simulink model "power_windgen"  (Simulink 6.0)
settings: Solver=ode23tb  StartTime=0.0  StopTime=5  RelTol=1e-4
InitFcn:
  | load power_windgen_init
undefined symbols (not defined in the file or in its folder): DiscIntNeverNeededParam, psbwindgen_char
libraries: powerlib x43, powerlib_extras x6
Description:
  | The Model initialization function Callback automatically
  | 
  | loads the initial states vector xInitial and the wind turbine
  | 
  | characteristics. The initial conditions are stored in the
  | 
  | power_windgen_init.mat file.
settings Model: Creator=Richard Gagnon, IREQ  LastModifiedBy=batserve  ExtModeAutoUpdateStatusClock=off  ProdHWDeviceType=Specified
settings DataIOCC: LimitDataPoints=off  LoadInitialState=on  SaveOutput=off  SignalLoggingName=sigsOut
settings OptimizationCC: BlockReduction=off  BooleanDataType=off
settings DebuggingCC: CheckExecutionContextPreStartOutputMsg=on  CheckExecutionContextRuntimeOutputMsg=on  SolverPrmCheckMsg=none
settings HardwareCC: ProdBitPerShort=32  ProdBitPerInt=16  ProdHWDeviceType=Specified  TargetUnknown=on

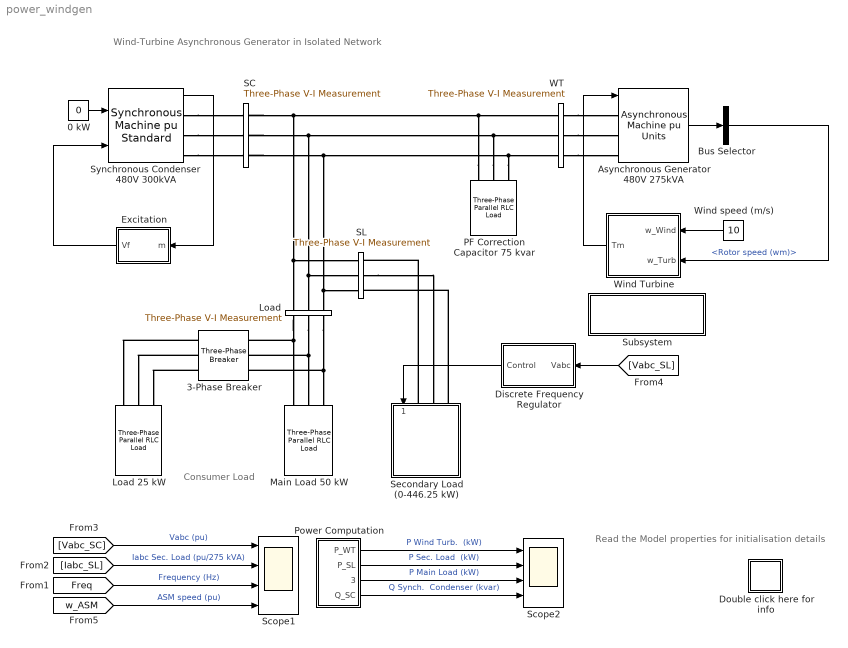
== system power_windgen ==
  note: Wind-Turbine Asynchronous Generator in Isolated Network
  note: Consumer Load
  note: Read the Model properties
      | for initialisation details
  0 kW : Constant  Value=0
  3-Phase Breaker : powerlib/Elements/Three-Phase Breaker  Orientation=left  InitialState=open  SwitchA=on  SwitchB=on  SwitchC=on  SwitchTimes=[0.2]  External=off  BreakerResistance=0.001  SnubberResistance=1e6  SnubberCapacitance=inf  Measurements=None
      settings: AttributesFormatString=\n
  Asynchronous Generator 480V 275kVA : powerlib/Machines/Asynchronous Machine pu Units  PresetModel=No  ShowDetailedParameters=on  RotorType=Squirrel-cage  ReferenceFrame=Rotor  NominalParameters=[ 275e3, 480, 60 ]  Stator=[ 0.016,0.06]  Rotor=[ 0.015,0.06]  Lm=3.5  Mechanical=[ 2,0,2 ]  InitialConditions=[-8.89496e-048 0 0.280896 0.280896 0.280896 -89.7425 150.258 30.2575]  Units=0  LoadFlowParameters=0
      settings: AttributesFormatString=\n
  Bus Selector : BusSelector  DialogController=Simulink.DDGSource_Bus  OutputSignals=Mechanical.Rotor speed (wm)
  Discrete Frequency Regulator : Subsystem  Orientation=left  mask(Discrete Frequency Regulator){Freq_ref=60, gains_regulator=[255 30], Vpp_nom=480, Ts=200e-6}
      mask prompts: Freq_ref "Reference frequency (Hz):"; gains_regulator "Regulator gains  [Kp Kd]:"; Vpp_nom "Phase to phase voltage (Vrms):"; Ts "Sample time (s):"
      mask help:
      | Input : phase to ground voltages
      |
      | Output : 24 logical signals for the control of the dump load
      mask init:
      | Vbase=Vpp_nom/sqrt(3);
      | Kp=gains_regulator(1);
      | Kd=gains_regulator(2);
  Double click here for info : Subsystem
      mask Display: disp('?')
  Excitation : Subsystem  Orientation=left
  Load : powerlib/Measurements/Three-Phase V-I Measurement  Orientation=down  VoltageMeasurement=phase-to-ground  SetLabelV=on  LabelV=Vabc_Load  Vpu=on  Vbase=480  CurrentMeasurement=yes  SetLabelI=on  LabelI=Iabc_Load  Ipu=on  Pbase=275e3  OutputType=Magnitude  PhasorSimulation=off  PSBequivalent=0
  Load 25 kW : powerlib/Elements/Three-Phase Parallel RLC Load  Orientation=down  PhysicalDomain=powersysdomain  SubClassName=unknown  LeftPortType=p1  RightPortType=p1  LConnTagsString=A|B|C  Configuration=Y (grounded)  NominalVoltage=480  NominalFrequency=60  ActivePower=25e3  InductivePower=0  CapacitivePower=0  Measurements=None
  Main Load 50 kW : powerlib/Elements/Three-Phase Parallel RLC Load  Orientation=down  PhysicalDomain=powersysdomain  SubClassName=unknown  LeftPortType=p1  RightPortType=p1  LConnTagsString=A|B|C  Configuration=Y (grounded)  NominalVoltage=480  NominalFrequency=60  ActivePower=50e3  InductivePower=0  CapacitivePower=0  Measurements=None
  PF Correction Capacitor 75 kvar : powerlib/Elements/Three-Phase Parallel RLC Load  Orientation=down  PhysicalDomain=powersysdomain  SubClassName=unknown  LeftPortType=p1  RightPortType=p1  LConnTagsString=A|B|C  Configuration=Delta  NominalVoltage=480  NominalFrequency=60  ActivePower=0  InductivePower=0  CapacitivePower=75e3  Measurements=None
  Power Computation : Subsystem
  SC : powerlib/Measurements/Three-Phase V-I Measurement  VoltageMeasurement=phase-to-ground  SetLabelV=on  LabelV=Vabc_SC  Vpu=on  Vbase=480  CurrentMeasurement=yes  SetLabelI=on  LabelI=Iabc_SC  Ipu=on  Pbase=300e3  OutputType=Magnitude  PhasorSimulation=off  PSBequivalent=0
  SL : powerlib/Measurements/Three-Phase V-I Measurement  VoltageMeasurement=phase-to-ground  SetLabelV=on  LabelV=Vabc_SL  Vpu=on  Vbase=480  CurrentMeasurement=yes  SetLabelI=on  LabelI=Iabc_SL  Ipu=on  Pbase=275e3  OutputType=Magnitude  PhasorSimulation=off  PSBequivalent=0
  Scope1 : Scope  NumInputPorts=4
      settings: TimeRange=5  YMin=-1.25~-0.75~59.8~1.008  YMax=1.25~0.75~60.1~1.013  SaveName=Vabc
  Scope2 : Scope  NumInputPorts=4
      settings: TimeRange=5  YMin=180~100~50~18  YMax=240~160~80~30  SaveName=Power  DataFormat=Array
  Secondary Load (0-446.25 kW) : Subsystem  Orientation=down  mask(8-step Variable Load){Vphase_phase_lissage=480, Freq=60, P_lissage_min=1.75e3, Pin_3phase=50e3}
      mask prompts: Vphase_phase_lissage "Nominal L-L voltage (Vrms):"; Freq "Nominal frequency (Hz):"; P_lissage_min "Power per step Pstep (W):"; Pin_3phase "Initial power  (W) :"
      mask help:
      | This block implements a variable, three-phase resistive load. The load variation uses an eight-bit binary progression so that the load power can be varied by steps from 0 to 255*Pstep.
      |
      | The eight three-phase resistors are connected in series with ideal switches simulating forced-commutated power electronic switches.
      |
      | The Pulses input is a vector containing the eight bits (0/1) controlling the eight three-phase switches. First value is the less significant bit.
      mask init:
      | Ron_switch=1e-6;
      | Rs_snubber=inf;
      | Cs_snubber=0;
      | n_niveaux=8;
      | Pmax=((2^n_niveaux)-1)*P_lissage_min;
      | Pin_normalise=min([(Pin_3phase/Pmax)*((2^n_niveaux)-1) ((2^n_niveaux)-1)]);
      | discret1=pow2(0:-1:-(n_niveaux-1))*Pin_normalise;
      | discret2=floor(discret1);
      | Status=rem(discret2,2);
  Subsystem : Subsystem
      settings: OpenFcn=open('psbwindgen_turb.fig')
      mask Display: disp('Double click to display\nTurbine characteristics')
  Synchronous Condenser  480V 300kVA : powerlib/Machines/Synchronous Machine pu Standard  PresetModel=No  ShowDetailedParameters=on  RotorType=Salient-pole  NominalParameters=[ 300e3 480 60 ]  Reactances1=[ 3.23, 0.21, 0.15, 2.79, 1.03, 0.37, 0.09 ]  Reactances2=[ 3.23, 0.21, 0.15, 2.79, 0.37, 0.09]  dAxisTimeConstants=Open-circuit  qAxisTimeConstants=Open-circuit  TimeConstants1="[ 1.7  0.008  0.004]"  TimeConstants2=[ 1.7, 0.008, 0.213, 0.004 ]  TimeConstants3="[  1.7 0.008 0.051266  ]"  TimeConstants4=[ 8.0, 0.03, 0.3371, 0.0295 ]  TimeConstants5="[ 0.08  0.019  0.004 ]"  TimeConstants6=[ 1.3201, 0.023, 1.0, 0.07 ]  TimeConstants7="[  0.08  0.019 0.051266  ]"  TimeConstants8=[ 1.3201, 0.0231, 0.3371, 0.0295 ]  StatorResistance=0.017  Mechanical=[ 1, 0, 2 ]  InitialConditions=[0 -89.2146 0.827 0.827 0.827 -86.4 153.6 33.6 2.71455]  SetSaturation=off  Saturation=[0.6404,0.7127,0.8441,0.9214,0.9956,1.082,1.19,1.316,1.457;0.7,0.7698,0.8872,0.9466,0.9969,1.046,1.1,1.151,1.201]  Units=0.5  LoadFlowParameters=[2 0 0 0 0]
      settings: AttributesFormatString=\n\n
  WT : powerlib/Measurements/Three-Phase V-I Measurement  VoltageMeasurement=phase-to-ground  SetLabelV=on  LabelV=Vabc_WT  Vpu=on  Vbase=480  CurrentMeasurement=yes  SetLabelI=on  LabelI=Iabc_WT  Ipu=on  Pbase=275e3  OutputType=Magnitude  PhasorSimulation=off  PSBequivalent=0
  Wind Turbine : Subsystem  Orientation=left
  Wind speed (m/s) : Constant  Orientation=left  Value=10
  wires:
  [Freq] -> Scope1/3  "Frequency (Hz)"
  [Vabc_SC] -> Scope1/1  "Vabc (pu)"
  [Iabc_SL] -> Scope1/2  "Iabc Sec. Load (pu/275 kVA)"
  Wind speed (m/s)/1 -> Wind Turbine/1(w_Wind)
  [Vabc_SL] -> Discrete Frequency Regulator/1(Vabc)
  Power Computation/1(P_WT) -> Scope2/1  "P Wind Turb.  (kW)"
  Power Computation/2(P_SL) -> Scope2/2  "P Sec. Load  (kW)"
  Power Computation/3(P_Load) -> Scope2/3  "P Main Load (kW)"
  Power Computation/4(Q_SC) -> Scope2/4  "Q Synch.  Condenser (kvar)"
  Discrete Frequency Regulator/1(Control) -> Secondary Load (0-446.25 kW)/1(Control)
  [w_ASM] -> Scope1/4  "ASM speed (pu)"
  0 kW/1 -> Synchronous Condenser  480V 300kVA/1
  Synchronous Condenser  480V 300kVA/1 -> Excitation/1(m)
  Excitation/1(Vf) -> Synchronous Condenser  480V 300kVA/2
  Asynchronous Generator 480V 275kVA/1 -> Bus Selector/1
  Wind Turbine/1(Tm) -> Asynchronous Generator 480V 275kVA/1
  Bus Selector/1 -> Wind Turbine/2(w_Turb)  "<Rotor speed (wm)>"
  connections:
  Load/RConn3 -- Main Load 50 kW/LConn3 -- 3-Phase Breaker/LConn3
  Load/RConn1 -- Main Load 50 kW/LConn1 -- 3-Phase Breaker/LConn1
  Load/RConn2 -- Main Load 50 kW/LConn2 -- 3-Phase Breaker/LConn2
  WT/RConn1 -- Asynchronous Generator 480V 275kVA/LConn1
  WT/RConn2 -- Asynchronous Generator 480V 275kVA/LConn2
  WT/RConn3 -- Asynchronous Generator 480V 275kVA/LConn3
  Synchronous Condenser  480V 300kVA/RConn1 -- SC/LConn1
  Synchronous Condenser  480V 300kVA/RConn2 -- SC/LConn2
  Synchronous Condenser  480V 300kVA/RConn3 -- SC/LConn3
  PF Correction Capacitor 75 kvar/LConn1 -- SC/RConn1 -- SL/LConn1 -- Load/LConn1 -- WT/LConn1
  PF Correction Capacitor 75 kvar/LConn2 -- SC/RConn2 -- SL/LConn2 -- Load/LConn2 -- WT/LConn2
  PF Correction Capacitor 75 kvar/LConn3 -- SC/RConn3 -- SL/LConn3 -- Load/LConn3 -- WT/LConn3
  3-Phase Breaker/RConn1 -- Load 25 kW/LConn1
  3-Phase Breaker/RConn2 -- Load 25 kW/LConn2
  3-Phase Breaker/RConn3 -- Load 25 kW/LConn3
  Secondary Load (0-446.25 kW)/LConn1 -- SL/RConn1
  SL/RConn2 -- Secondary Load (0-446.25 kW)/LConn2
  Secondary Load (0-446.25 kW)/LConn3 -- SL/RConn3

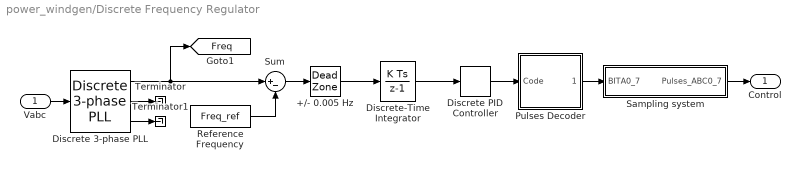
== system power_windgen/Discrete Frequency Regulator ==
  Vabc : Inport  Port=1  LatchInput=off
  +/- 0.005 Hz : DeadZone  LowerValue=-0.005  UpperValue=0.005  SaturateOnIntegerOverflow=on
  Discrete 3-phase PLL : powerlib_extras/Discrete  Control Blocks/Discrete 3-phase PLL  Fmin=45  Par_Init=[0 Freq_ref]  ParK=[60 1400]  Ts=Ts
  Discrete PID Controller : powerlib_extras/Discrete  Control Blocks/Discrete PID Controller  Kp=Kp  Ki=0  Kd=Kd  TcD=0.5e-3  Par_Limits=[255 0]  Init=0  Ts=Ts
  Discrete-Time Integrator : DiscreteIntegrator  SampleTime=Ts  LimitOutput=on  UpperSaturationLimit=1  LowerSaturationLimit=0  ICPrevOutput=DiscIntNeverNeededParam  ICPrevScaledInput=DiscIntNeverNeededParam
  Pulses Decoder : Subsystem  mask(Pulses Decoder){n=8}
      mask prompts: n "Number of bits to decode:"
      mask help:
      | Decode the scalar input 'Code' into a vector output 'Pulses' based on  the specified number of bits to decode.
      | (Element 1 of vector output = least significant bit)
  Reference Frequency : Constant  Value=Freq_ref
  Sampling system : Subsystem
  Sum : Sum  Inputs=|+-  SaturateOnIntegerOverflow=on  InputSameDT=on
  Terminator : Terminator
  Terminator1 : Terminator
  Control : Outport
  tag scope: Freq=global
  wires:
  Vabc/1 -> Discrete 3-phase PLL/1
  Discrete 3-phase PLL/3 -> Terminator1/1
  Discrete 3-phase PLL/2 -> Terminator/1
  Sampling system/1(Pulses_ABC0_7) -> Control/1
  Discrete-Time Integrator/1 -> Discrete PID Controller/1
  Reference Frequency/1 -> Sum/2
  Discrete PID Controller/1 -> Pulses Decoder/1(Code)
  Sum/1 -> +/- 0.005 Hz/1
  Pulses Decoder/1(Pulses) -> Sampling system/1(BITA0_7)
  +/- 0.005 Hz/1 -> Discrete-Time Integrator/1
  Discrete 3-phase PLL/1 -> Sum/1, [Freq]

== system power_windgen/Double click here for info ==
  note: [1] R. Gagnon, B. Saulnier, G. Sybille, P. Giroux; "Modeling of a Generic High-Penetration No-Storage Wind-Diesel System Using Matlab/Power System Blockset"
      | 2002 Global Windpower Conference, April 2002, Paris, France
      | [2] B. Saulnier, A.O. Barry, B. Dube, R. Reid; "Design and Development of a Regulation and Control System for the High-Penetration No-Storage Wind/Diesel
      | Scheme" European Community Wind Energy Conference 88, 6-10 june 1988, Herning, Denmark
      | [3] L. Mott (NPS), B. Saulnier (IREQ) " Commercial Wind-Diesel Project, St. Paul Island, Alaska" 14th Prime Power Diesel Inter-Utility Conference,
      | May 28-June 2, Winnipeg, Manitoba, Canada
  note: References
  note: For the demo, the wind speed (10m/s) is such that the wind turbine produces enough power to supply the load. The diesel-generator (not simulated) is stopped
      | and the synchronous machine operates as a synchronous condenser with its mechanical power input (Pm) set at zero.
      | The demo illustrates the dynamic performance of the frequency regulation system when an additional 25 kW customer load is switched on.
      |
      | Start simulation and observe voltages, currents, powers, asynchronous machine speed and system frequency on the two scopes.
      | Initial conditions (xInitial vector) have been automatically loaded in your workspace so that simulation starts in steady state.
      |
      | As the asynchronous machine operates in generator mode, its speed is slightly above the synchronous speed (1.011 pu).
      | According to turbine characteristics, for a 10m/s wind speed, the turbine output power is 0.75 pu (206 kW). Because of the asynchronous machine losses,
      | the wind turbine produces 200 kW. As the main load is 50 kW, the secondary load absorbs 150 kW to maintain a constant 60 Hz frequency.
      | At t=0.2 s, the additional load of 25 kW is switched on. The frequency  momentarily drops to 59.85 Hz and the frequency regulator reacts to reduce the power
      | absorbed by the secondary load in order to bring the frequency back to 60 Hz. Voltage stays at 1 pu and no flicker is observed.
  note: R. Reid, B. Saulnier, R. Gagnon; Hydro-Quebec (IREQ)
  note: A generic model of the High-Penetration, No Storage, Wind-Diesel (HPNSWD) system is presented in this demo [1].
      | This technology was developed by Hydro-Quebec to reduce the cost of supplying electricity in remote northern communities[2].
      | The optimal wind penetration (installed wind capacity/peak electrical demand) for this system depends on the site delivery cost of fuel
      | and available wind resource. The first commercial application of HPNSWD technology was commissioned in 1999 by Northern Power Systems (Vermont,USA)
      | on St. Paul Island, Alaska [3]. The HPNSWD system presented in this demo uses a 480 V, 300 kVA synchronous machine, a wind turbine driving
      | a 480 V, 275 kVA induction generator, a 50 kW customer load and a variable secondary load (0 to 446.25 kW).
      |
      | At low wind speeds both the induction generator and the diesel-driven synchronous generator are required to feed the load.
      | When the wind power exceeds the load demand, it is possible to shut down the diesel-generator. In this all-wind mode, the synchronous machine
      | is used as a synchronous condenser and its excitation system controls the grid voltage at its nominal value.
      | A secondary load bank is used to regulate the system frequency by absorbing the wind power exceeding consumer demand.
      |
      | The Wind Turbine block uses a 2-D Lookup Table to compute the turbine torque output (Tm) as a function of wind speed (w_Wind) and turbine speed (w_Turb).
      | When you opened this demo, the Pm(w_Wind, w_Turb) characteristics was automatically loaded in your workspace (psbwindgen_char array).
      | To display the turbine characteristics, double click on the block located below the Wind Turbine block.
      |
      | The Secondary Load block consists of eight sets of three-phase resistors connected in series with GTO thyristor switches.
      | The nominal power of each set follows a binary progression so that the load can be varied from 0 to 446.25 kW by steps of 1.75kW.
      | GTOs are simulated by ideal switches.
      |
      | The frequency is controlled by the Discrete Frequency Regulator block. This controller uses a standard three-phase Phase Locked Loop (PLL) system to
      | measure the system frequency. The measured frequency is compared to the reference frequency (60 Hz) to obtain the frequency error.
      | This error is integrated to obtain the phase error. The phase error is then used  by a Proportional-Differential (PD) controller to produce an output signal
      | representing the required secondary load power. This signal is converted to an 8-bit digital signal controlling switching of the eight three-phase secondary loads.
      | In order to minimize voltage disturbances, switching is performed at zero crossing of voltage.
  note: Wind-Turbine Asynchronous Generator in Isolated Network
  note: Circuit Description
  note: Demonstration

== system power_windgen/Excitation ==
  m : Inport  Orientation=left  Port=1  LatchInput=off
  Bus Selector1 : BusSelector  Orientation=left  DialogController=Simulink.DDGSource_Bus  OutputSignals="dq0 components.Stator voltage  vd (pu),dq0 components.Stator voltage  vq (pu)"
  Constant3 : Constant  Orientation=left
  Excitation System : powerlib/Machines/Excitation System  Orientation=left  tr=20e-3  reg=[ 300, 0.001 ]  exc=[ 1, 0 ]  tgr=[ 0, 0 ]  damp=[ 0.001, 0.1 ]  sat=[ 0, 0 ]  lim=[ -11.5, 11.5, 0 ]  v0=[1,2.71455]
  Ground : Ground  Orientation=left
  Vf : Outport  Orientation=left
  wires:
  Constant3/1 -> Excitation System/1
  Ground/1 -> Excitation System/4
  m/1 -> Bus Selector1/1
  Excitation System/1 -> Vf/1
  Bus Selector1/1 -> Excitation System/2  "<Stator voltage  vd (pu)>"
  Bus Selector1/2 -> Excitation System/3  "<Stator voltage  vq (pu)>"

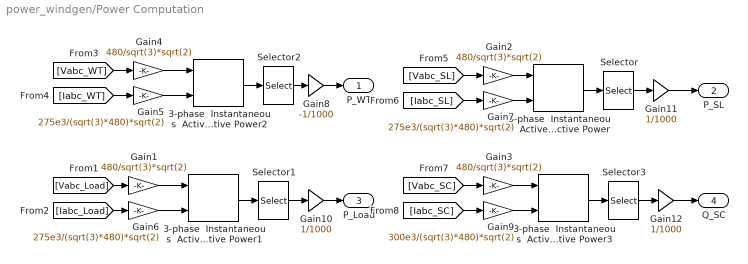
== system power_windgen/Power Computation ==
  3-phase  Instantaneous  Active & Reactive Power{,1..3} (4 alike) : powerlib_extras/Measurements/3-phase  Instantaneous  Active & Reactive Power
  Gain{1..4} (4 alike) : Gain  Gain=480/sqrt(3)*sqrt(2)  SaturateOnIntegerOverflow=on
  Gain10 : Gain  Gain=1/1000  SaturateOnIntegerOverflow=on
  Gain11 : Gain  Gain=1/1000  SaturateOnIntegerOverflow=on
  Gain12 : Gain  Gain=1/1000  SaturateOnIntegerOverflow=on
  Gain5 : Gain  Gain=275e3/(sqrt(3)*480)*sqrt(2)  SaturateOnIntegerOverflow=on
  Gain6 : Gain  Gain=275e3/(sqrt(3)*480)*sqrt(2)  SaturateOnIntegerOverflow=on
  Gain7 : Gain  Gain=275e3/(sqrt(3)*480)*sqrt(2)  SaturateOnIntegerOverflow=on
  Gain8 : Gain  Gain=-1/1000  SaturateOnIntegerOverflow=on
  Gain9 : Gain  Gain=300e3/(sqrt(3)*480)*sqrt(2)  SaturateOnIntegerOverflow=on
  Selector : Selector  Elements=[1]  InputPortWidth=2
  Selector1 : Selector  Elements=[1]  InputPortWidth=2
  Selector2 : Selector  Elements=[1]  InputPortWidth=2
  Selector3 : Selector  Elements=[2]  InputPortWidth=2
  P_WT : Outport
  P_SL : Outport  Port=2
  P_Load : Outport  Port=3
  Q_SC : Outport  Port=4
  wires:
  3-phase  Instantaneous  Active & Reactive Power/1 -> Selector/1
  Selector/1 -> Gain11/1
  3-phase  Instantaneous  Active & Reactive Power1/1 -> Selector1/1
  3-phase  Instantaneous  Active & Reactive Power2/1 -> Selector2/1
  [Vabc_WT] -> Gain4/1
  [Iabc_WT] -> Gain5/1
  3-phase  Instantaneous  Active & Reactive Power3/1 -> Selector3/1
  Gain4/1 -> 3-phase  Instantaneous  Active & Reactive Power2/1
  Gain5/1 -> 3-phase  Instantaneous  Active & Reactive Power2/2
  [Vabc_Load] -> Gain1/1
  [Iabc_Load] -> Gain6/1
  Gain1/1 -> 3-phase  Instantaneous  Active & Reactive Power1/1
  Gain6/1 -> 3-phase  Instantaneous  Active & Reactive Power1/2
  [Vabc_SL] -> Gain2/1
  [Iabc_SL] -> Gain7/1
  Gain2/1 -> 3-phase  Instantaneous  Active & Reactive Power/1
  Gain7/1 -> 3-phase  Instantaneous  Active & Reactive Power/2
  Selector1/1 -> Gain10/1
  Selector2/1 -> Gain8/1
  Gain8/1 -> P_WT/1
  Selector3/1 -> Gain12/1
  [Vabc_SC] -> Gain3/1
  [Iabc_SC] -> Gain9/1
  Gain3/1 -> 3-phase  Instantaneous  Active & Reactive Power3/1
  Gain9/1 -> 3-phase  Instantaneous  Active & Reactive Power3/2
  Gain10/1 -> P_Load/1
  Gain11/1 -> P_SL/1
  Gain12/1 -> Q_SC/1

== system power_windgen/Secondary Load (0-446.25 kW) ==
  Control : Inport  Port=1  LatchInput=off
  Demux : Demux  Outputs=8
  Resistive Loads : Subsystem
  Switches : Subsystem
  A : PMIOPort  Port=1  Side=Left
  B : PMIOPort  Port=2  Side=Left
  C : PMIOPort  Port=3  Side=Left
  wires:
  Control/1 -> Demux/1
  Demux/8 -> Switches/8(P_ABC7)
  Demux/7 -> Switches/7(P_ABC6)
  Demux/6 -> Switches/6(P_ABC5)
  Demux/5 -> Switches/5(P_ABC4)
  Demux/4 -> Switches/4(P_ABC3)
  Demux/3 -> Switches/3(P_ABC2)
  Demux/2 -> Switches/2(P_ABC1)
  Demux/1 -> Switches/1(P_ABC0)
  connections:
  Switches/RConn1 -- Resistive Loads/LConn1
  Switches/RConn2 -- Resistive Loads/LConn2
  Switches/RConn3 -- Resistive Loads/LConn3
  Switches/RConn4 -- Resistive Loads/LConn4
  Switches/RConn5 -- Resistive Loads/LConn5
  Switches/RConn6 -- Resistive Loads/LConn6
  Switches/RConn7 -- Resistive Loads/LConn7
  Switches/RConn8 -- Resistive Loads/LConn8
  Switches/RConn9 -- Resistive Loads/LConn9
  Switches/RConn10 -- Resistive Loads/LConn10
  Switches/RConn11 -- Resistive Loads/LConn11
  Switches/RConn12 -- Resistive Loads/LConn12
  Switches/RConn13 -- Resistive Loads/LConn13
  Switches/RConn14 -- Resistive Loads/LConn14
  Switches/RConn15 -- Resistive Loads/LConn15
  Switches/RConn16 -- Resistive Loads/LConn16
  Switches/RConn17 -- Resistive Loads/LConn17
  Switches/RConn18 -- Resistive Loads/LConn18
  Switches/RConn19 -- Resistive Loads/LConn19
  Switches/RConn20 -- Resistive Loads/LConn20
  Switches/RConn21 -- Resistive Loads/LConn21
  Switches/RConn22 -- Resistive Loads/LConn22
  Switches/RConn23 -- Resistive Loads/LConn23
  Switches/RConn24 -- Resistive Loads/LConn24
  A/RConn1 -- Switches/LConn1
  B/RConn1 -- Switches/LConn2
  C/RConn1 -- Switches/LConn3

== system power_windgen/Subsystem ==

== system power_windgen/Wind Turbine ==
  w_Wind : Inport  Port=1  LatchInput=off
  w_Turb : Inport  Port=2  LatchInput=off
  1800 rpm : Gain  Gain=1800  SaturateOnIntegerOverflow=on
  Constant3 : Constant  Value=1e-6
  Gain : Gain  Gain=-1  SaturateOnIntegerOverflow=on
  P(w_Wind,w_Turb) : Lookup2D  DialogController=Simulink.DDGSource  RowIndex=[0 5 6 7 8 9 10 11 12]  ColumnIndex=[0 571.55 685.8 800.15 914.4 1028.8 1143.1 1257.4 1371.7 1486 1600.3 1714.6 1828.9 1943.2 2057.5 2171.8 2286.1 2400.5 2514.7 2629.1 2743.3 2857.7 2971.9 3086.3 3200.5 3314.9 3429.2]  OutputValues=psbwindgen_char  SaturateOnIntegerOverflow=on  InputSameDT=on
  Product : Product  Inputs=*/  SaturateOnIntegerOverflow=on  InputSameDT=on
  Switch : Switch  Threshold=1e-6  SaturateOnIntegerOverflow=on  InputSameDT=on
  Tm : Outport
  tag scope: w_ASM=global
  wires:
  w_Turb/1 -> 1800 rpm/1, Switch/1, Switch/2, [w_ASM]
  Constant3/1 -> Switch/3
  w_Wind/1 -> P(w_Wind,w_Turb)/1
  P(w_Wind,w_Turb)/1 -> Product/1
  Switch/1 -> Product/2
  Product/1 -> Gain/1
  Gain/1 -> Tm/1
  1800 rpm/1 -> P(w_Wind,w_Turb)/2

== system power_windgen/Discrete Frequency Regulator/Pulses Decoder ==
  Code : Inport  Port=1  LatchInput=off
  Constant : Constant  Value=pow2(0:-1:-(n-1))
  Constant6 : Constant  Value=2
  Math Function : Math  Operator=rem  SaturateOnIntegerOverflow=on
  Product : Product  SaturateOnIntegerOverflow=on  InputSameDT=on
  Rounding Function : Rounding
  Pulses : Outport
  wires:
  Math Function/1 -> Pulses/1
  Rounding Function/1 -> Math Function/1
  Constant6/1 -> Math Function/2
  Product/1 -> Rounding Function/1
  Code/1 -> Product/1
  Constant/1 -> Product/2

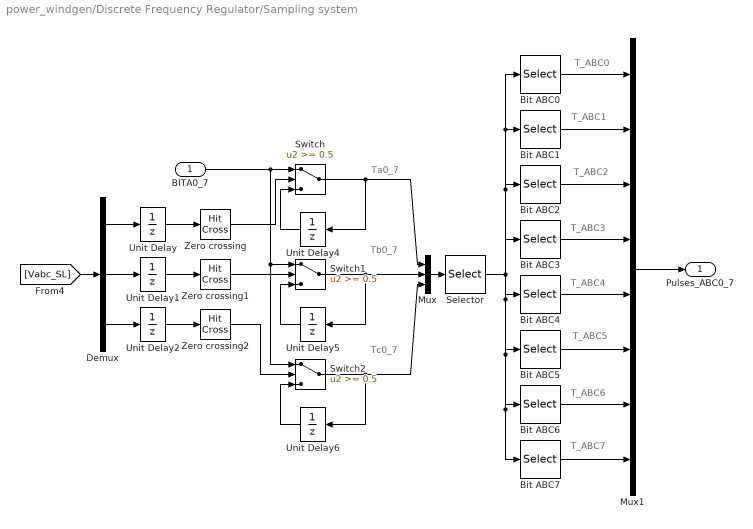
== system power_windgen/Discrete Frequency Regulator/Sampling system ==
  note: T_ABC7
  note: T_ABC6
  note: T_ABC5
  note: T_ABC4
  note: T_ABC3
  note: T_ABC2
  note: T_ABC1
  note: T_ABC0
  note: Tc0_7
  note: Tb0_7
  note: Ta0_7
  BITA0_7 : Inport  Port=1  LatchInput=off
  " Bit ABC4" : Selector  Elements=[13 14 15]  InputPortWidth=24
  Bit ABC0 : Selector  Elements=[1 2 3]  InputPortWidth=24
  Bit ABC1 : Selector  Elements=[4 5 6]  InputPortWidth=24
  Bit ABC2 : Selector  Elements=[7 8 9]  InputPortWidth=24
  Bit ABC3 : Selector  Elements=[10 11 12]  InputPortWidth=24
  Bit ABC5 : Selector  Elements=[16 17 18]  InputPortWidth=24
  Bit ABC6 : Selector  Elements=[19 20 21]  InputPortWidth=24
  Bit ABC7 : Selector  Elements=[22 23 24]  InputPortWidth=24
  Demux : Demux  Outputs=3
  Mux : Mux  Inputs=3
  Mux1 : Mux  Inputs=8
  Selector : Selector  Elements=[1 9 17 2 10 18 3 11 19 4 12 20 5 13 21 6 14 22 7 15 23 8 16 24]  InputPortWidth=24
  Switch : Switch  Threshold=0.5  SaturateOnIntegerOverflow=on  InputSameDT=on
  Switch1 : Switch  Threshold=0.5  SaturateOnIntegerOverflow=on  InputSameDT=on
  Switch2 : Switch  Threshold=0.5  SaturateOnIntegerOverflow=on  InputSameDT=on
  Unit Delay : UnitDelay  SampleTime=Ts
  Unit Delay1 : UnitDelay  SampleTime=Ts
  Unit Delay2 : UnitDelay  SampleTime=Ts
  Unit Delay4 : UnitDelay  Orientation=left  SampleTime=Ts
  Unit Delay5 : UnitDelay  Orientation=left  SampleTime=Ts
  Unit Delay6 : UnitDelay  Orientation=left  SampleTime=Ts
  Zero crossing : HitCross
  Zero crossing1 : HitCross
  Zero crossing2 : HitCross
  Pulses_ABC0_7 : Outport
  wires:
  BITA0_7/1 -> Switch2/1, Switch1/1, Switch/1
  Demux/3 -> Unit Delay2/1
  Demux/2 -> Unit Delay1/1
  Demux/1 -> Unit Delay/1
  Mux1/1 -> Pulses_ABC0_7/1
  Bit ABC7/1 -> Mux1/8
  Bit ABC6/1 -> Mux1/7
  Bit ABC5/1 -> Mux1/6
  " Bit ABC4"/1 -> Mux1/5
  Bit ABC3/1 -> Mux1/4
  Bit ABC2/1 -> Mux1/3
  Bit ABC1/1 -> Mux1/2
  Bit ABC0/1 -> Mux1/1
  Selector/1 -> Bit ABC7/1, Bit ABC6/1, Bit ABC5/1, " Bit ABC4"/1, Bit ABC3/1, Bit ABC2/1, Bit ABC0/1, Bit ABC1/1
  Mux/1 -> Selector/1
  Unit Delay6/1 -> Switch2/3
  Switch2/1 -> Mux/3, Unit Delay6/1
  Unit Delay5/1 -> Switch1/3
  Switch1/1 -> Mux/2, Unit Delay5/1
  Unit Delay4/1 -> Switch/3
  Switch/1 -> Mux/1, Unit Delay4/1
  Unit Delay/1 -> Zero crossing/1
  Unit Delay2/1 -> Zero crossing2/1
  Zero crossing/1 -> Switch/2
  Zero crossing1/1 -> Switch1/2
  Zero crossing2/1 -> Switch2/2
  [Vabc_SL] -> Demux/1
  Unit Delay1/1 -> Zero crossing1/1

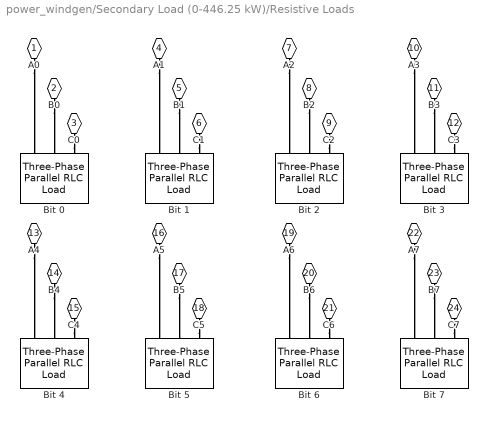
== system power_windgen/Secondary Load (0-446.25 kW)/Resistive Loads ==
  Bit 0 : powerlib/Elements/Three-Phase Parallel RLC Load  Orientation=down  PhysicalDomain=powersysdomain  SubClassName=unknown  LeftPortType=p1  RightPortType=p1  LConnTagsString=A|B|C  Configuration=Y (grounded)  NominalVoltage=Vphase_phase_lissage  NominalFrequency=Freq  ActivePower=P_lissage_min  InductivePower=0  CapacitivePower=0  Measurements=None
  Bit 1 : powerlib/Elements/Three-Phase Parallel RLC Load  Orientation=down  PhysicalDomain=powersysdomain  SubClassName=unknown  LeftPortType=p1  RightPortType=p1  LConnTagsString=A|B|C  Configuration=Y (grounded)  NominalVoltage=Vphase_phase_lissage  NominalFrequency=Freq  ActivePower=2*P_lissage_min  InductivePower=0  CapacitivePower=0  Measurements=None
  Bit 2 : powerlib/Elements/Three-Phase Parallel RLC Load  Orientation=down  PhysicalDomain=powersysdomain  SubClassName=unknown  LeftPortType=p1  RightPortType=p1  LConnTagsString=A|B|C  Configuration=Y (grounded)  NominalVoltage=Vphase_phase_lissage  NominalFrequency=Freq  ActivePower=2^2*P_lissage_min  InductivePower=0  CapacitivePower=0  Measurements=None
  Bit 3 : powerlib/Elements/Three-Phase Parallel RLC Load  Orientation=down  PhysicalDomain=powersysdomain  SubClassName=unknown  LeftPortType=p1  RightPortType=p1  LConnTagsString=A|B|C  Configuration=Y (grounded)  NominalVoltage=Vphase_phase_lissage  NominalFrequency=Freq  ActivePower=2^3*P_lissage_min  InductivePower=0  CapacitivePower=0  Measurements=None
  Bit 4 : powerlib/Elements/Three-Phase Parallel RLC Load  Orientation=down  PhysicalDomain=powersysdomain  SubClassName=unknown  LeftPortType=p1  RightPortType=p1  LConnTagsString=A|B|C  Configuration=Y (grounded)  NominalVoltage=Vphase_phase_lissage  NominalFrequency=Freq  ActivePower=2^4*P_lissage_min  InductivePower=0  CapacitivePower=0  Measurements=None
  Bit 5 : powerlib/Elements/Three-Phase Parallel RLC Load  Orientation=down  PhysicalDomain=powersysdomain  SubClassName=unknown  LeftPortType=p1  RightPortType=p1  LConnTagsString=A|B|C  Configuration=Y (grounded)  NominalVoltage=Vphase_phase_lissage  NominalFrequency=Freq  ActivePower=2^5*P_lissage_min  InductivePower=0  CapacitivePower=0  Measurements=None
  Bit 6 : powerlib/Elements/Three-Phase Parallel RLC Load  Orientation=down  PhysicalDomain=powersysdomain  SubClassName=unknown  LeftPortType=p1  RightPortType=p1  LConnTagsString=A|B|C  Configuration=Y (grounded)  NominalVoltage=Vphase_phase_lissage  NominalFrequency=Freq  ActivePower=2^6*P_lissage_min  InductivePower=0  CapacitivePower=0  Measurements=None
  Bit 7 : powerlib/Elements/Three-Phase Parallel RLC Load  Orientation=down  PhysicalDomain=powersysdomain  SubClassName=unknown  LeftPortType=p1  RightPortType=p1  LConnTagsString=A|B|C  Configuration=Y (grounded)  NominalVoltage=Vphase_phase_lissage  NominalFrequency=Freq  ActivePower=2^7*P_lissage_min  InductivePower=0  CapacitivePower=0  Measurements=None
  A0 : PMIOPort  Orientation=down  Port=1  Side=Left
  B0 : PMIOPort  Orientation=down  Port=2  Side=Left
  C0 : PMIOPort  Orientation=down  Port=3  Side=Left
  A1 : PMIOPort  Orientation=down  Port=4  Side=Left
  B1 : PMIOPort  Orientation=down  Port=5  Side=Left
  C1 : PMIOPort  Orientation=down  Port=6  Side=Left
  A2 : PMIOPort  Orientation=down  Port=7  Side=Left
  B2 : PMIOPort  Orientation=down  Port=8  Side=Left
  C2 : PMIOPort  Orientation=down  Port=9  Side=Left
  A3 : PMIOPort  Orientation=down  Port=10  Side=Left
  B3 : PMIOPort  Orientation=down  Port=11  Side=Left
  C3 : PMIOPort  Orientation=down  Port=12  Side=Left
  A4 : PMIOPort  Orientation=down  Port=13  Side=Left
  B4 : PMIOPort  Orientation=down  Port=14  Side=Left
  C4 : PMIOPort  Orientation=down  Port=15  Side=Left
  A5 : PMIOPort  Orientation=down  Port=16  Side=Left
  B5 : PMIOPort  Orientation=down  Port=17  Side=Left
  C5 : PMIOPort  Orientation=down  Port=18  Side=Left
  A6 : PMIOPort  Orientation=down  Port=19  Side=Left
  B6 : PMIOPort  Orientation=down  Port=20  Side=Left
  C6 : PMIOPort  Orientation=down  Port=21  Side=Left
  A7 : PMIOPort  Orientation=down  Port=22  Side=Left
  B7 : PMIOPort  Orientation=down  Port=23  Side=Left
  C7 : PMIOPort  Orientation=down  Port=24  Side=Left
  connections:
  C7/RConn1 -- Bit 7/LConn3
  B7/RConn1 -- Bit 7/LConn2
  A7/RConn1 -- Bit 7/LConn1
  C6/RConn1 -- Bit 6/LConn3
  B6/RConn1 -- Bit 6/LConn2
  A6/RConn1 -- Bit 6/LConn1
  C5/RConn1 -- Bit 5/LConn3
  B5/RConn1 -- Bit 5/LConn2
  A5/RConn1 -- Bit 5/LConn1
  C4/RConn1 -- Bit 4/LConn3
  B4/RConn1 -- Bit 4/LConn2
  A4/RConn1 -- Bit 4/LConn1
  C3/RConn1 -- Bit 3/LConn3
  B3/RConn1 -- Bit 3/LConn2
  A3/RConn1 -- Bit 3/LConn1
  C2/RConn1 -- Bit 2/LConn3
  B2/RConn1 -- Bit 2/LConn2
  A2/RConn1 -- Bit 2/LConn1
  C1/RConn1 -- Bit 1/LConn3
  B1/RConn1 -- Bit 1/LConn2
  A1/RConn1 -- Bit 1/LConn1
  C0/RConn1 -- Bit 0/LConn3
  B0/RConn1 -- Bit 0/LConn2
  A0/RConn1 -- Bit 0/LConn1

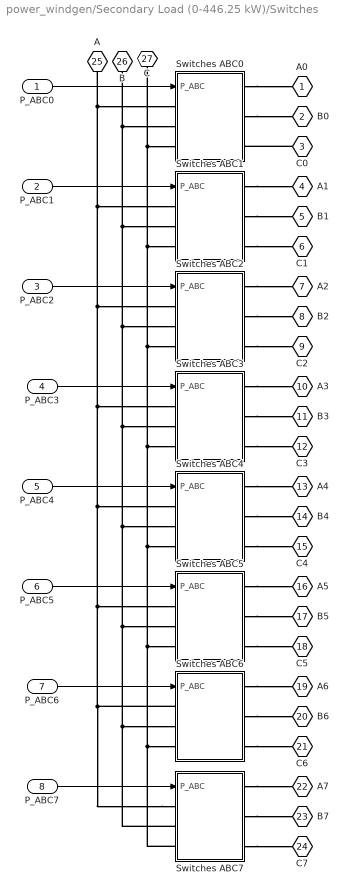
== system power_windgen/Secondary Load (0-446.25 kW)/Switches ==
  P_ABC0 : Inport  Port=1  LatchInput=off
  P_ABC1 : Inport  Port=2  LatchInput=off
  P_ABC2 : Inport  Port=3  LatchInput=off
  P_ABC3 : Inport  Port=4  LatchInput=off
  P_ABC4 : Inport  Port=5  LatchInput=off
  P_ABC5 : Inport  Port=6  LatchInput=off
  P_ABC6 : Inport  Port=7  LatchInput=off
  P_ABC7 : Inport  Port=8  LatchInput=off
  Switches ABC0 : Subsystem
  Switches ABC1 : Subsystem
  Switches ABC2 : Subsystem
  Switches ABC3 : Subsystem
  Switches ABC4 : Subsystem
  Switches ABC5 : Subsystem
  Switches ABC6 : Subsystem
  Switches ABC7 : Subsystem
  A0 : PMIOPort  Orientation=left  Port=1  Side=Right
  B0 : PMIOPort  Orientation=left  Port=2  Side=Right
  C0 : PMIOPort  Orientation=left  Port=3  Side=Right
  A1 : PMIOPort  Orientation=left  Port=4  Side=Right
  B1 : PMIOPort  Orientation=left  Port=5  Side=Right
  C1 : PMIOPort  Orientation=left  Port=6  Side=Right
  A2 : PMIOPort  Orientation=left  Port=7  Side=Right
  B2 : PMIOPort  Orientation=left  Port=8  Side=Right
  C2 : PMIOPort  Orientation=left  Port=9  Side=Right
  A3 : PMIOPort  Orientation=left  Port=10  Side=Right
  B3 : PMIOPort  Orientation=left  Port=11  Side=Right
  C3 : PMIOPort  Orientation=left  Port=12  Side=Right
  A4 : PMIOPort  Orientation=left  Port=13  Side=Right
  B4 : PMIOPort  Orientation=left  Port=14  Side=Right
  C4 : PMIOPort  Orientation=left  Port=15  Side=Right
  A5 : PMIOPort  Orientation=left  Port=16  Side=Right
  B5 : PMIOPort  Orientation=left  Port=17  Side=Right
  C5 : PMIOPort  Orientation=left  Port=18  Side=Right
  A6 : PMIOPort  Orientation=left  Port=19  Side=Right
  B6 : PMIOPort  Orientation=left  Port=20  Side=Right
  C6 : PMIOPort  Orientation=left  Port=21  Side=Right
  A7 : PMIOPort  Orientation=left  Port=22  Side=Right
  B7 : PMIOPort  Orientation=left  Port=23  Side=Right
  C7 : PMIOPort  Orientation=left  Port=24  Side=Right
  A : PMIOPort  Orientation=down  Port=25  Side=Left
  B : PMIOPort  Orientation=down  Port=26  Side=Left
  C : PMIOPort  Orientation=down  Port=27  Side=Left
  wires:
  P_ABC7/1 -> Switches ABC7/1(P_ABC)
  P_ABC6/1 -> Switches ABC6/1(P_ABC)
  P_ABC5/1 -> Switches ABC5/1(P_ABC)
  P_ABC4/1 -> Switches ABC4/1(P_ABC)
  P_ABC3/1 -> Switches ABC3/1(P_ABC)
  P_ABC2/1 -> Switches ABC2/1(P_ABC)
  P_ABC1/1 -> Switches ABC1/1(P_ABC)
  P_ABC0/1 -> Switches ABC0/1(P_ABC)
  connections:
  Switches ABC0/RConn1 -- A0/RConn1
  Switches ABC0/RConn2 -- B0/RConn1
  C0/RConn1 -- Switches ABC0/RConn3
  Switches ABC1/RConn1 -- A1/RConn1
  Switches ABC1/RConn2 -- B1/RConn1
  Switches ABC1/RConn3 -- C1/RConn1
  Switches ABC2/RConn1 -- A2/RConn1
  Switches ABC2/RConn2 -- B2/RConn1
  Switches ABC2/RConn3 -- C2/RConn1
  Switches ABC3/RConn1 -- A3/RConn1
  Switches ABC3/RConn2 -- B3/RConn1
  Switches ABC3/RConn3 -- C3/RConn1
  Switches ABC4/RConn1 -- A4/RConn1
  Switches ABC4/RConn2 -- B4/RConn1
  Switches ABC4/RConn3 -- C4/RConn1
  Switches ABC5/RConn1 -- A5/RConn1
  Switches ABC5/RConn2 -- B5/RConn1
  Switches ABC5/RConn3 -- C5/RConn1
  Switches ABC6/RConn1 -- A6/RConn1
  Switches ABC6/RConn2 -- B6/RConn1
  Switches ABC6/RConn3 -- C6/RConn1
  Switches ABC7/RConn3 -- C7/RConn1
  Switches ABC7/RConn2 -- B7/RConn1
  Switches ABC7/RConn1 -- A7/RConn1
  Switches ABC7/LConn2 -- Switches ABC0/LConn2 -- B/RConn1 -- Switches ABC1/LConn2 -- Switches ABC2/LConn2 -- Switches ABC3/LConn2 -- Switches ABC4/LConn2 -- Switches ABC5/LConn2 -- Switches ABC6/LConn2
  Switches ABC7/LConn3 -- Switches ABC0/LConn3 -- C/RConn1 -- Switches ABC1/LConn3 -- Switches ABC2/LConn3 -- Switches ABC3/LConn3 -- Switches ABC4/LConn3 -- Switches ABC5/LConn3 -- Switches ABC6/LConn3
  Switches ABC7/LConn1 -- Switches ABC0/LConn1 -- A/RConn1 -- Switches ABC1/LConn1 -- Switches ABC2/LConn1 -- Switches ABC3/LConn1 -- Switches ABC4/LConn1 -- Switches ABC5/LConn1 -- Switches ABC6/LConn1

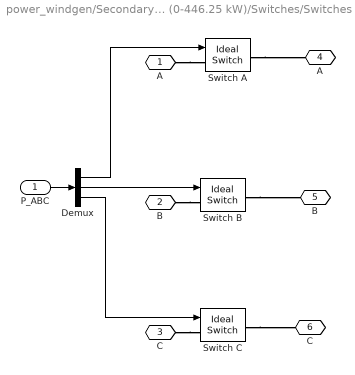
== system power_windgen/Secondary Load (0-446.25 kW)/Switches/Switches ABC0 ==
  P_ABC : Inport  Port=1  LatchInput=off
  Demux : Demux  Outputs=3
  Switch A : powerlib/Power Electronics/Ideal Switch  Ron=Ron_switch  Lon=0  IC=Status(1)  Rs=Rs_snubber  Cs=Cs_snubber  Measurements=off
      settings: AttributesFormatString=\n
  Switch B : powerlib/Power Electronics/Ideal Switch  Ron=Ron_switch  Lon=0  IC=Status(1)  Rs=Rs_snubber  Cs=Cs_snubber  Measurements=off
      settings: AttributesFormatString=\n
  Switch C : powerlib/Power Electronics/Ideal Switch  Ron=Ron_switch  Lon=0  IC=Status(1)  Rs=Rs_snubber  Cs=Cs_snubber  Measurements=off
      settings: AttributesFormatString=\n
  A : PMIOPort  Port=1  Side=Left
  B : PMIOPort  Port=2  Side=Left
  C : PMIOPort  Port=3  Side=Left
  "A " : PMIOPort  Orientation=left  Port=4  Side=Right
  "B " : PMIOPort  Orientation=left  Port=5  Side=Right
  "C " : PMIOPort  Orientation=left  Port=6  Side=Right
  wires:
  P_ABC/1 -> Demux/1
  Demux/3 -> Switch C/1
  Demux/2 -> Switch B/1
  Demux/1 -> Switch A/1
  connections:
  Switch C/RConn1 -- "C "/RConn1
  Switch B/RConn1 -- "B "/RConn1
  Switch A/RConn1 -- "A "/RConn1
  C/RConn1 -- Switch C/LConn1
  B/RConn1 -- Switch B/LConn1
  A/RConn1 -- Switch A/LConn1

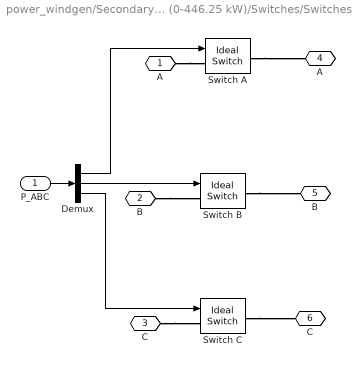
== system power_windgen/Secondary Load (0-446.25 kW)/Switches/Switches ABC1 ==
  P_ABC : Inport  Port=1  LatchInput=off
  Demux : Demux  Outputs=3
  Switch A : powerlib/Power Electronics/Ideal Switch  Ron=Ron_switch  Lon=0  IC=Status(2)  Rs=Rs_snubber  Cs=Cs_snubber  Measurements=off
      settings: AttributesFormatString=\n
  Switch B : powerlib/Power Electronics/Ideal Switch  Ron=Ron_switch  Lon=0  IC=Status(2)  Rs=Rs_snubber  Cs=Cs_snubber  Measurements=off
      settings: AttributesFormatString=\n
  Switch C : powerlib/Power Electronics/Ideal Switch  Ron=Ron_switch  Lon=0  IC=Status(2)  Rs=Rs_snubber  Cs=Cs_snubber  Measurements=off
      settings: AttributesFormatString=\n
  A : PMIOPort  Port=1  Side=Left
  B : PMIOPort  Port=2  Side=Left
  C : PMIOPort  Port=3  Side=Left
  "A " : PMIOPort  Orientation=left  Port=4  Side=Right
  "B " : PMIOPort  Orientation=left  Port=5  Side=Right
  "C " : PMIOPort  Orientation=left  Port=6  Side=Right
  wires:
  Demux/1 -> Switch A/1
  Demux/2 -> Switch B/1
  Demux/3 -> Switch C/1
  P_ABC/1 -> Demux/1
  connections:
  A/RConn1 -- Switch A/LConn1
  B/RConn1 -- Switch B/LConn1
  Switch A/RConn1 -- "A "/RConn1
  Switch B/RConn1 -- "B "/RConn1
  Switch C/RConn1 -- "C "/RConn1
  C/RConn1 -- Switch C/LConn1

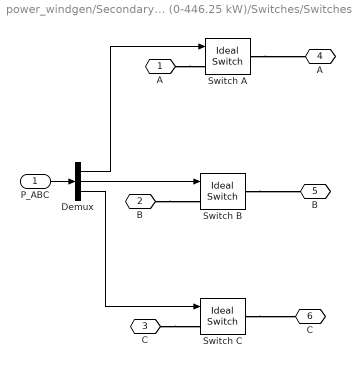
== system power_windgen/Secondary Load (0-446.25 kW)/Switches/Switches ABC2 ==
  P_ABC : Inport  Port=1  LatchInput=off
  Demux : Demux  Outputs=3
  Switch A : powerlib/Power Electronics/Ideal Switch  Ron=Ron_switch  Lon=0  IC=Status(3)  Rs=Rs_snubber  Cs=Cs_snubber  Measurements=off
      settings: AttributesFormatString=\n
  Switch B : powerlib/Power Electronics/Ideal Switch  Ron=Ron_switch  Lon=0  IC=Status(3)  Rs=Rs_snubber  Cs=Cs_snubber  Measurements=off
      settings: AttributesFormatString=\n
  Switch C : powerlib/Power Electronics/Ideal Switch  Ron=Ron_switch  Lon=0  IC=Status(3)  Rs=Rs_snubber  Cs=Cs_snubber  Measurements=off
      settings: AttributesFormatString=\n
  A : PMIOPort  Port=1  Side=Left
  B : PMIOPort  Port=2  Side=Left
  C : PMIOPort  Port=3  Side=Left
  "A " : PMIOPort  Orientation=left  Port=4  Side=Right
  "B " : PMIOPort  Orientation=left  Port=5  Side=Right
  "C " : PMIOPort  Orientation=left  Port=6  Side=Right
  wires:
  P_ABC/1 -> Demux/1
  Demux/3 -> Switch C/1
  Demux/2 -> Switch B/1
  Demux/1 -> Switch A/1
  connections:
  Switch C/RConn1 -- "C "/RConn1
  Switch B/RConn1 -- "B "/RConn1
  Switch A/RConn1 -- "A "/RConn1
  A/RConn1 -- Switch A/LConn1
  B/RConn1 -- Switch B/LConn1
  C/RConn1 -- Switch C/LConn1

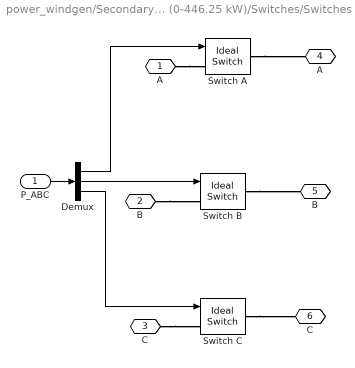
== system power_windgen/Secondary Load (0-446.25 kW)/Switches/Switches ABC3 ==
  P_ABC : Inport  Port=1  LatchInput=off
  Demux : Demux  Outputs=3
  Switch A : powerlib/Power Electronics/Ideal Switch  Ron=Ron_switch  Lon=0  IC=Status(4)  Rs=Rs_snubber  Cs=Cs_snubber  Measurements=off
      settings: AttributesFormatString=\n
  Switch B : powerlib/Power Electronics/Ideal Switch  Ron=Ron_switch  Lon=0  IC=Status(4)  Rs=Rs_snubber  Cs=Cs_snubber  Measurements=off
      settings: AttributesFormatString=\n
  Switch C : powerlib/Power Electronics/Ideal Switch  Ron=Ron_switch  Lon=0  IC=Status(4)  Rs=Rs_snubber  Cs=Cs_snubber  Measurements=off
      settings: AttributesFormatString=\n
  A : PMIOPort  Port=1  Side=Left
  B : PMIOPort  Port=2  Side=Left
  C : PMIOPort  Port=3  Side=Left
  "A " : PMIOPort  Orientation=left  Port=4  Side=Right
  "B " : PMIOPort  Orientation=left  Port=5  Side=Right
  "C " : PMIOPort  Orientation=left  Port=6  Side=Right
  wires:
  Demux/1 -> Switch A/1
  Demux/2 -> Switch B/1
  Demux/3 -> Switch C/1
  P_ABC/1 -> Demux/1
  connections:
  C/RConn1 -- Switch C/LConn1
  B/RConn1 -- Switch B/LConn1
  A/RConn1 -- Switch A/LConn1
  Switch A/RConn1 -- "A "/RConn1
  Switch B/RConn1 -- "B "/RConn1
  Switch C/RConn1 -- "C "/RConn1

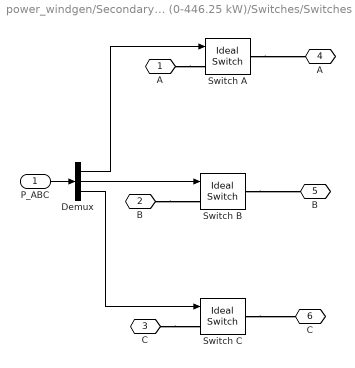
== system power_windgen/Secondary Load (0-446.25 kW)/Switches/Switches ABC4 ==
  P_ABC : Inport  Port=1  LatchInput=off
  Demux : Demux  Outputs=3
  Switch A : powerlib/Power Electronics/Ideal Switch  Ron=Ron_switch  Lon=0  IC=Status(5)  Rs=Rs_snubber  Cs=Cs_snubber  Measurements=off
      settings: AttributesFormatString=\n
  Switch B : powerlib/Power Electronics/Ideal Switch  Ron=Ron_switch  Lon=0  IC=Status(5)  Rs=Rs_snubber  Cs=Cs_snubber  Measurements=off
      settings: AttributesFormatString=\n
  Switch C : powerlib/Power Electronics/Ideal Switch  Ron=Ron_switch  Lon=0  IC=Status(5)  Rs=Rs_snubber  Cs=Cs_snubber  Measurements=off
      settings: AttributesFormatString=\n
  A : PMIOPort  Port=1  Side=Left
  B : PMIOPort  Port=2  Side=Left
  C : PMIOPort  Port=3  Side=Left
  "A " : PMIOPort  Orientation=left  Port=4  Side=Right
  "B " : PMIOPort  Orientation=left  Port=5  Side=Right
  "C " : PMIOPort  Orientation=left  Port=6  Side=Right
  wires:
  P_ABC/1 -> Demux/1
  Demux/3 -> Switch C/1
  Demux/2 -> Switch B/1
  Demux/1 -> Switch A/1
  connections:
  Switch C/RConn1 -- "C "/RConn1
  Switch B/RConn1 -- "B "/RConn1
  Switch A/RConn1 -- "A "/RConn1
  A/RConn1 -- Switch A/LConn1
  B/RConn1 -- Switch B/LConn1
  C/RConn1 -- Switch C/LConn1

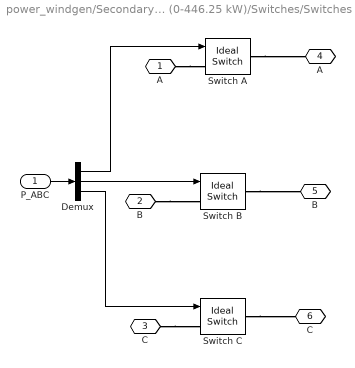
== system power_windgen/Secondary Load (0-446.25 kW)/Switches/Switches ABC5 ==
  P_ABC : Inport  Port=1  LatchInput=off
  Demux : Demux  Outputs=3
  Switch A : powerlib/Power Electronics/Ideal Switch  Ron=Ron_switch  Lon=0  IC=Status(6)  Rs=Rs_snubber  Cs=Cs_snubber  Measurements=off
      settings: AttributesFormatString=\n
  Switch B : powerlib/Power Electronics/Ideal Switch  Ron=Ron_switch  Lon=0  IC=Status(6)  Rs=Rs_snubber  Cs=Cs_snubber  Measurements=off
      settings: AttributesFormatString=\n
  Switch C : powerlib/Power Electronics/Ideal Switch  Ron=Ron_switch  Lon=0  IC=Status(6)  Rs=Rs_snubber  Cs=Cs_snubber  Measurements=off
      settings: AttributesFormatString=\n
  A : PMIOPort  Port=1  Side=Left
  B : PMIOPort  Port=2  Side=Left
  C : PMIOPort  Port=3  Side=Left
  "A " : PMIOPort  Orientation=left  Port=4  Side=Right
  "B " : PMIOPort  Orientation=left  Port=5  Side=Right
  "C " : PMIOPort  Orientation=left  Port=6  Side=Right
  wires:
  Demux/1 -> Switch A/1
  Demux/2 -> Switch B/1
  Demux/3 -> Switch C/1
  P_ABC/1 -> Demux/1
  connections:
  C/RConn1 -- Switch C/LConn1
  B/RConn1 -- Switch B/LConn1
  A/RConn1 -- Switch A/LConn1
  Switch A/RConn1 -- "A "/RConn1
  Switch B/RConn1 -- "B "/RConn1
  Switch C/RConn1 -- "C "/RConn1

== system power_windgen/Secondary Load (0-446.25 kW)/Switches/Switches ABC6 ==
  P_ABC : Inport  Port=1  LatchInput=off
  Demux : Demux  Outputs=3
  Switch A : powerlib/Power Electronics/Ideal Switch  Ron=Ron_switch  Lon=0  IC=Status(7)  Rs=Rs_snubber  Cs=Cs_snubber  Measurements=off
      settings: AttributesFormatString=\n
  Switch B : powerlib/Power Electronics/Ideal Switch  Ron=Ron_switch  Lon=0  IC=Status(7)  Rs=Rs_snubber  Cs=Cs_snubber  Measurements=off
      settings: AttributesFormatString=\n
  Switch C : powerlib/Power Electronics/Ideal Switch  Ron=Ron_switch  Lon=0  IC=Status(7)  Rs=Rs_snubber  Cs=Cs_snubber  Measurements=off
      settings: AttributesFormatString=\n
  A : PMIOPort  Port=1  Side=Left
  B : PMIOPort  Port=2  Side=Left
  C : PMIOPort  Port=3  Side=Left
  "A " : PMIOPort  Orientation=left  Port=4  Side=Right
  "B " : PMIOPort  Orientation=left  Port=5  Side=Right
  "C " : PMIOPort  Orientation=left  Port=6  Side=Right
  wires:
  P_ABC/1 -> Demux/1
  Demux/3 -> Switch C/1
  Demux/2 -> Switch B/1
  Demux/1 -> Switch A/1
  connections:
  Switch C/RConn1 -- "C "/RConn1
  Switch B/RConn1 -- "B "/RConn1
  Switch A/RConn1 -- "A "/RConn1
  A/RConn1 -- Switch A/LConn1
  B/RConn1 -- Switch B/LConn1
  C/RConn1 -- Switch C/LConn1

== system power_windgen/Secondary Load (0-446.25 kW)/Switches/Switches ABC7 ==
  P_ABC : Inport  Port=1  LatchInput=off
  Demux : Demux  Outputs=3
  Switch A : powerlib/Power Electronics/Ideal Switch  Ron=Ron_switch  Lon=0  IC=Status(8)  Rs=Rs_snubber  Cs=Cs_snubber  Measurements=off
      settings: AttributesFormatString=\n
  Switch B : powerlib/Power Electronics/Ideal Switch  Ron=Ron_switch  Lon=0  IC=Status(8)  Rs=Rs_snubber  Cs=Cs_snubber  Measurements=off
      settings: AttributesFormatString=\n
  Switch C : powerlib/Power Electronics/Ideal Switch  Ron=Ron_switch  Lon=0  IC=Status(8)  Rs=Rs_snubber  Cs=Cs_snubber  Measurements=off
      settings: AttributesFormatString=\n
  A : PMIOPort  Port=1  Side=Left
  B : PMIOPort  Port=2  Side=Left
  C : PMIOPort  Port=3  Side=Left
  "A " : PMIOPort  Orientation=left  Port=4  Side=Right
  "B " : PMIOPort  Orientation=left  Port=5  Side=Right
  "C " : PMIOPort  Orientation=left  Port=6  Side=Right
  wires:
  Demux/1 -> Switch A/1
  Demux/2 -> Switch B/1
  Demux/3 -> Switch C/1
  P_ABC/1 -> Demux/1
  connections:
  C/RConn1 -- Switch C/LConn1
  B/RConn1 -- Switch B/LConn1
  A/RConn1 -- Switch A/LConn1
  Switch A/RConn1 -- "A "/RConn1
  Switch B/RConn1 -- "B "/RConn1
  Switch C/RConn1 -- "C "/RConn1
